simulink model "test_config"  (R2024b)
settings: Solver=VariableStepAuto  StartTime=0.0  StopTime=10.0  RelTol=1e-3
settings Model: Creator=rcmas  LastModifiedBy=rcmas

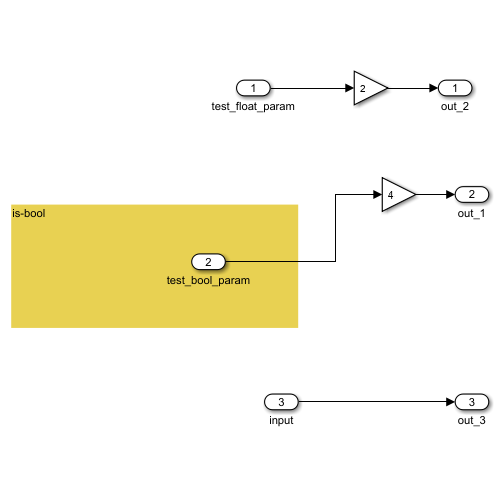
[thumbnail: Simulink's stored preview of the top-level diagram]
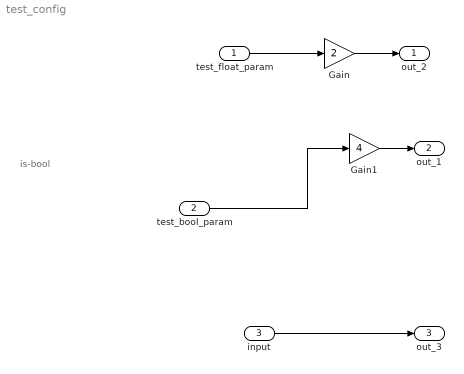
== system test_config ==
  note: is-bool
  test_float_param : Inport
  test_bool_param : Inport  Port=2
  input : Inport  Port=3
  Gain : Gain  Gain=2
  Gain1 : Gain  Gain=4
  out_2 : Outport
  out_1 : Outport  Port=2
  out_3 : Outport  Port=3
  wires:
  test_float_param/1 -> Gain/1
  Gain/1 -> out_2/1
  test_bool_param/1 -> Gain1/1
  Gain1/1 -> out_1/1
  input/1 -> out_3/1
